simulink model "Task1"  (R2023a)
settings: Solver=VariableStepAuto  StartTime=0.0  StopTime=10.0  RelTol=1e-3
settings Model: Creator=MUHAMMAD SADEEQ  LastModifiedBy=MUHAMMAD SADEEQ

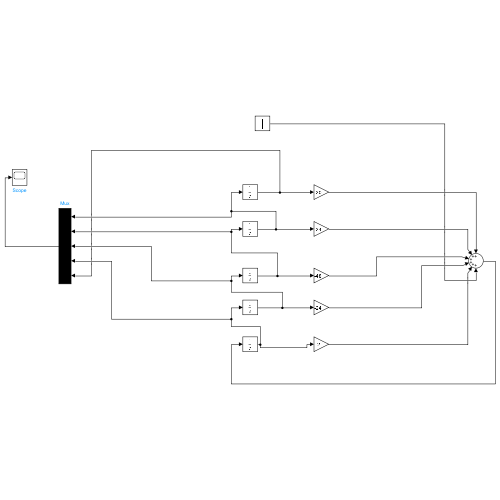
[thumbnail: Simulink's stored preview of the top-level diagram]
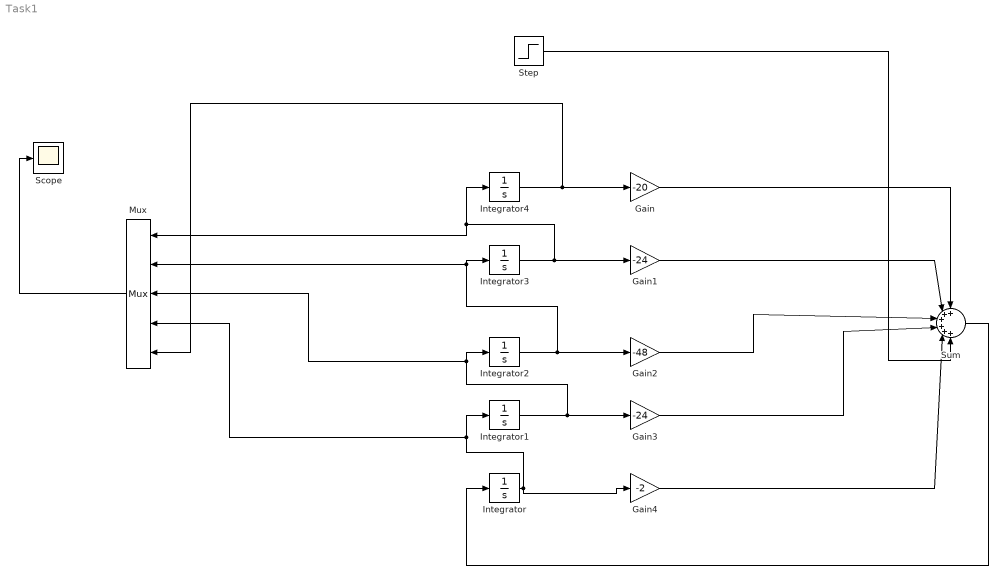
== system Task1 ==
  Gain : Gain  Gain=-20
  Gain1 : Gain  Gain=-24
  Gain2 : Gain  Gain=-48
  Gain3 : Gain  Gain=-24
  Gain4 : Gain  Gain=-2
  Integrator{,1..4} (5 alike) : Integrator
  Mux : Mux  Inputs=5
  Scope : Scope
  Step : Step  After=10  SampleTime=0
  Sum : Sum  Inputs=++++++
  wires:
  Gain/1 -> Sum/1
  Gain1/1 -> Sum/2
  Gain2/1 -> Sum/3
  Gain3/1 -> Sum/4
  Gain4/1 -> Sum/5
  Sum/1 -> Integrator/1
  Integrator/1 -> Mux/4, Integrator1/1, Gain4/1
  Integrator1/1 -> Mux/3, Integrator2/1, Gain3/1
  Integrator2/1 -> Mux/2, Integrator3/1, Gain2/1
  Integrator3/1 -> Integrator4/1, Mux/1, Gain1/1
  Integrator4/1 -> Mux/5, Gain/1
  Mux/1 -> Scope/1
  Step/1 -> Sum/6
